simulink model "PFC_PID_Control_2_"  (R2025a)
settings: Solver=ode23tb  StartTime=0.0  StopTime=0.1  FixedStep=1e-06  MaxStep=1e-5  RelTol=1e-4  AbsTol=1e-6
undefined symbols (not defined in the file or in its folder): I_pk
libraries: slpidlib x2
settings Model: Creator=kesav  LastModifiedBy=kesav

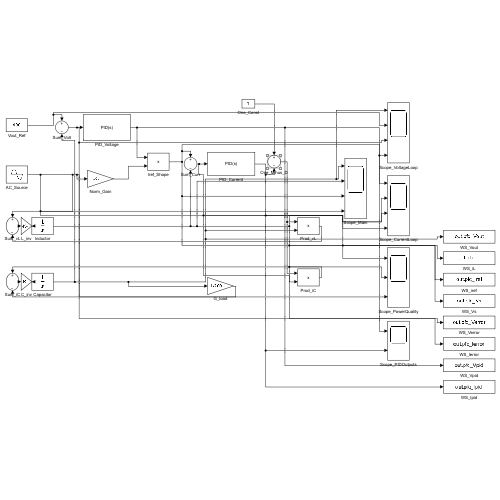
[thumbnail: Simulink's stored preview of the top-level diagram]
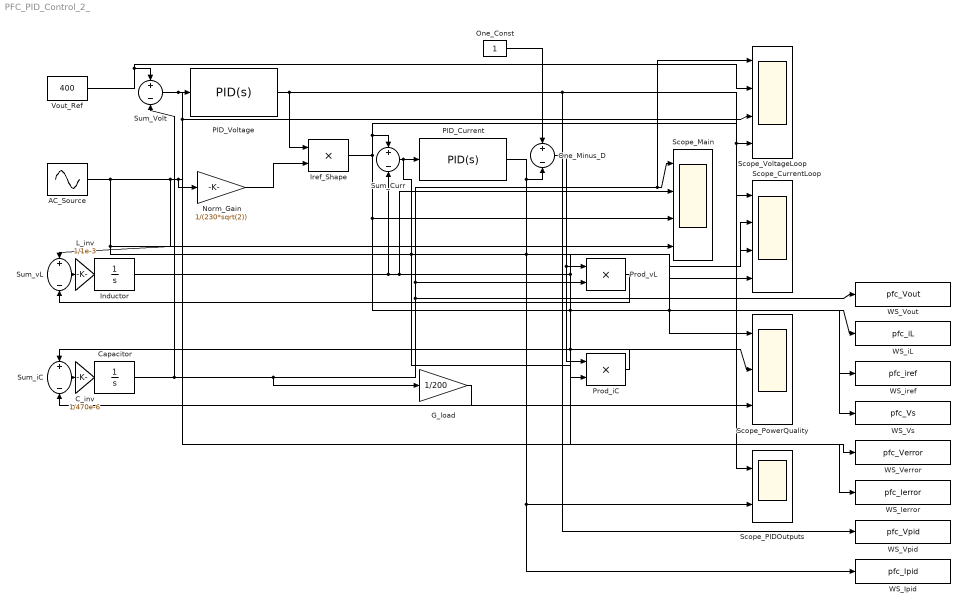
== system PFC_PID_Control_2_ ==
  AC_Source : Sin  Amplitude=325.27  Frequency=2*pi*50  SampleTime=0
  C_inv : Gain  Gain=1/470e-6
  Capacitor : Integrator
  G_load : Gain  Gain=1/200
  Inductor : Integrator
  Iref_Shape : Product
  L_inv : Gain  Gain=1/1e-3
  Norm_Gain : Gain  Gain=1/(230*sqrt(2))
  One_Const : Constant
  One_Minus_D : Sum  Inputs=+-
  PID_Current : slpidlib/PID Controller  Controller=PID  Form=Parallel  TimeDomain=Continuous-time  UseExternalTs=off  SampleTime=-1  IntegratorMethod=Forward Euler  FilterMethod=Forward Euler  ControllerParametersSource=internal  P=0.5  I=50  UseKiTs=off  D=0  UseExternalDerivativeSource=off  N=100  UseFilter=on  TunerSelectOption=Transfer Function Based (PID Tuner App)  InitialConditionSource=internal  InitialConditionForIntegrator=0  InitialConditionForFilter=0  DifferentiatorICPrevScaledInput=0  ExternalReset=none  TrackingMode=off  Kt=1  LimitOutput=off  SatLimitsSource=internal  UpperSaturationLimit=0.95  LowerSaturationLimit=-0.95  LinearizeAsGain=on  AntiWindupMode=clamping  Kb=1  LimitIntegrator=off  UpperIntegratorSaturationLimit=inf  LowerIntegratorSaturationLimit=-inf  POutMin=[]  POutMax=[]  IOutMin=[]  IOutMax=[]  DOutMin=[]  DOutMax=[]  NOutMin=[]  NOutMax=[]  SumOutMin=[]  SumOutMax=[]  SaturationOutMin=[]  SaturationOutMax=[]  PParamMin=[]  PParamMax=[]  IParamMin=[]  IParamMax=[]  DParamMin=[]  DParamMax=[]  NParamMin=[]  NParamMax=[]  KbParamMin=[]  KbParamMax=[]  KtParamMin=[]  KtParamMax=[]  KbOutMin=[]  KbOutMax=[]  KtOutMin=[]  KtOutMax=[]  IntegratorOutMin=[]  IntegratorOutMax=[]  FilterOutMin=[]  FilterOutMax=[]  SumI1OutMin=[]  SumI1OutMax=[]  SumI2OutMin=[]  SumI2OutMax=[]  SumI3OutMin=[]  SumI3OutMax=[]  SumI4OutMin=[]  SumI4OutMax=[]  SumDOutMin=[]  SumDOutMax=[]  DifferentiatorOutMin=[]  DifferentiatorOutMax=[]  FilterDiffOutCoefMin=[]  FilterDiffOutCoefMax=[]  ReciprocalOutMin=[]  ReciprocalOutMax=[]  SumDenOutMin=[]  SumDenOutMax=[]  SumNumOutMin=[]  SumNumOutMax=[]  DivideOutMin=[]  DivideOutMax=[]  UdiffTsProdOutMin=[]  UdiffTsProdOutMax=[]  NTsProdOutMin=[]  NTsProdOutMax=[]  UintegralTsProdOutMin=[]  UintegralTsProdOutMax=[]  UngainTsProdOutMin=[]  UngainTsProdOutMax=[]  ClampingZeroOutDataTypeStr=Inherit: Inherit via back propagation  ClampingZeroOutMin=[]  ClampingZeroOutMax=[]  FilterDenConstantOutDataTypeStr=Inherit: Inherit via back propagation  FilterDenConstantOutMin=[]  FilterDenConstantOutMax=[]  PCopyOutDataTypeStr=Inherit: Inherit via back propagation  PCopyOutMin=[]  PCopyOutMax=[]  NCopyOutDataTypeStr=Inherit: Inherit via back propagation  NCopyOutMin=[]  NCopyOutMax=[]  IntegratorContinuousStateAttributes=''  IntegratorStateMustResolveToSignalObject=off  IntegratorRTWStateStorageClass=Auto  FilterContinuousStateAttributes=''  FilterStateMustResolveToSignalObject=off  FilterRTWStateStorageClass=Auto  ParallelPVariant=InternalParameters  IdealPVariant=Disabled  IVariant=InternalParameters  DVariant=InternalParameters  IntegratorVariant=Continuous  SatVariant=Disabled  AWVariant=Passthrough  PCopyVariant=Disabled  TRVariant=Disabled  FdbkBlocksVariant=Forward  IdealPFdbkVariant=Disabled  SatFdbkVariant=Disabled  DerivativeFilterVariant=ContFilter  NVariant=InternalParameters  NCopyVariant=Disabled  FilterICVariant=InternalICsFilter  IntegratorICVariant=InternalICs  ExternalResetVariant=Disabled  TRSumVariant=Passthrough  SumFdbkVariant=Disabled  SumVariant=Sum_PID  TsampFilterVariant=InternalTs  TsampNgainVariant=Passthrough  TsampIntegralVariant=Disabled_SignalSpec  ExternalSaturationOutDataTypeStr=Inherit: Same as second input  DerivativeSourceVariant=ErrorSignal  PreIntVariant=InternalPreInt
  PID_Voltage : slpidlib/PID Controller  Controller=PID  Form=Parallel  TimeDomain=Continuous-time  UseExternalTs=off  SampleTime=-1  IntegratorMethod=Forward Euler  FilterMethod=Forward Euler  ControllerParametersSource=internal  P=0.3  I=20  UseKiTs=off  D=0  UseExternalDerivativeSource=off  N=10  UseFilter=on  TunerSelectOption=Transfer Function Based (PID Tuner App)  InitialConditionSource=internal  InitialConditionForIntegrator=0  InitialConditionForFilter=0  DifferentiatorICPrevScaledInput=0  ExternalReset=none  TrackingMode=off  Kt=1  LimitOutput=off  SatLimitsSource=internal  UpperSaturationLimit=I_pk  LowerSaturationLimit=0  LinearizeAsGain=on  AntiWindupMode=clamping  Kb=1  LimitIntegrator=off  UpperIntegratorSaturationLimit=inf  LowerIntegratorSaturationLimit=-inf  POutMin=[]  POutMax=[]  IOutMin=[]  IOutMax=[]  DOutMin=[]  DOutMax=[]  NOutMin=[]  NOutMax=[]  SumOutMin=[]  SumOutMax=[]  SaturationOutMin=[]  SaturationOutMax=[]  PParamMin=[]  PParamMax=[]  IParamMin=[]  IParamMax=[]  DParamMin=[]  DParamMax=[]  NParamMin=[]  NParamMax=[]  KbParamMin=[]  KbParamMax=[]  KtParamMin=[]  KtParamMax=[]  KbOutMin=[]  KbOutMax=[]  KtOutMin=[]  KtOutMax=[]  IntegratorOutMin=[]  IntegratorOutMax=[]  FilterOutMin=[]  FilterOutMax=[]  SumI1OutMin=[]  SumI1OutMax=[]  SumI2OutMin=[]  SumI2OutMax=[]  SumI3OutMin=[]  SumI3OutMax=[]  SumI4OutMin=[]  SumI4OutMax=[]  SumDOutMin=[]  SumDOutMax=[]  DifferentiatorOutMin=[]  DifferentiatorOutMax=[]  FilterDiffOutCoefMin=[]  FilterDiffOutCoefMax=[]  ReciprocalOutMin=[]  ReciprocalOutMax=[]  SumDenOutMin=[]  SumDenOutMax=[]  SumNumOutMin=[]  SumNumOutMax=[]  DivideOutMin=[]  DivideOutMax=[]  UdiffTsProdOutMin=[]  UdiffTsProdOutMax=[]  NTsProdOutMin=[]  NTsProdOutMax=[]  UintegralTsProdOutMin=[]  UintegralTsProdOutMax=[]  UngainTsProdOutMin=[]  UngainTsProdOutMax=[]  ClampingZeroOutDataTypeStr=Inherit: Inherit via back propagation  ClampingZeroOutMin=[]  ClampingZeroOutMax=[]  FilterDenConstantOutDataTypeStr=Inherit: Inherit via back propagation  FilterDenConstantOutMin=[]  FilterDenConstantOutMax=[]  PCopyOutDataTypeStr=Inherit: Inherit via back propagation  PCopyOutMin=[]  PCopyOutMax=[]  NCopyOutDataTypeStr=Inherit: Inherit via back propagation  NCopyOutMin=[]  NCopyOutMax=[]  IntegratorContinuousStateAttributes=''  IntegratorStateMustResolveToSignalObject=off  IntegratorRTWStateStorageClass=Auto  FilterContinuousStateAttributes=''  FilterStateMustResolveToSignalObject=off  FilterRTWStateStorageClass=Auto  ParallelPVariant=InternalParameters  IdealPVariant=Disabled  IVariant=InternalParameters  DVariant=InternalParameters  IntegratorVariant=Continuous  SatVariant=Disabled  AWVariant=Passthrough  PCopyVariant=Disabled  TRVariant=Disabled  FdbkBlocksVariant=Forward  IdealPFdbkVariant=Disabled  SatFdbkVariant=Disabled  DerivativeFilterVariant=ContFilter  NVariant=InternalParameters  NCopyVariant=Disabled  FilterICVariant=InternalICsFilter  IntegratorICVariant=InternalICs  ExternalResetVariant=Disabled  TRSumVariant=Passthrough  SumFdbkVariant=Disabled  SumVariant=Sum_PID  TsampFilterVariant=InternalTs  TsampNgainVariant=Passthrough  TsampIntegralVariant=Disabled_SignalSpec  ExternalSaturationOutDataTypeStr=Inherit: Same as second input  DerivativeSourceVariant=ErrorSignal  PreIntVariant=InternalPreInt
  Prod_iC : Product
  Prod_vL : Product
  Scope_CurrentLoop : Scope  NumInputPorts=4
      settings: ActiveDisplayYMinimum=-45.830688238369063  ActiveDisplayYMaximum=53.057681548956552
  Scope_Main : Scope  NumInputPorts=4
  Scope_PIDOutputs : Scope  NumInputPorts=2
      settings: ActiveDisplayYMinimum=-1  ActiveDisplayYMaximum=1
  Scope_PowerQuality : Scope  NumInputPorts=3
      settings: ActiveDisplayYMinimum=-1  ActiveDisplayYMaximum=1
  Scope_VoltageLoop : Scope  NumInputPorts=4
  Sum_Curr : Sum  Inputs=+-
  Sum_Volt : Sum  Inputs=+-
  Sum_iC : Sum  Inputs=+-
  Sum_vL : Sum  Inputs=+-
  Vout_Ref : Constant  Value=400
  WS_Ierror : ToWorkspace  VariableName=pfc_Ierror  SampleTime=-1
  WS_Ipid : ToWorkspace  VariableName=pfc_Ipid  SampleTime=-1
  WS_Verror : ToWorkspace  VariableName=pfc_Verror  SampleTime=-1
  WS_Vout : ToWorkspace  VariableName=pfc_Vout  SampleTime=-1
  WS_Vpid : ToWorkspace  VariableName=pfc_Vpid  SampleTime=-1
  WS_Vs : ToWorkspace  VariableName=pfc_Vs  SampleTime=-1
  WS_iL : ToWorkspace  VariableName=pfc_iL  SampleTime=-1
  WS_iref : ToWorkspace  VariableName=pfc_iref  SampleTime=-1
  wires:
  Vout_Ref/1 -> Sum_Volt/1, Scope_VoltageLoop/2
  AC_Source/1 -> Norm_Gain/1, Scope_PowerQuality/3, Sum_vL/1, Scope_PowerQuality/1, WS_Vs/1, Scope_Main/4
  PID_Voltage/1 -> Scope_VoltageLoop/4, Scope_PIDOutputs/1, WS_Vpid/1, Iref_Shape/1
  Norm_Gain/1 -> Iref_Shape/2
  Iref_Shape/1 -> Scope_Main/3, WS_iref/1, Sum_Curr/1, Scope_CurrentLoop/1
  Prod_vL/1 -> Sum_vL/2
  Sum_vL/1 -> L_inv/1
  L_inv/1 -> Inductor/1
  Prod_iC/1 -> Sum_iC/1
  G_load/1 -> Sum_iC/2
  Sum_iC/1 -> C_inv/1
  C_inv/1 -> Capacitor/1
  One_Const/1 -> One_Minus_D/1
  PID_Current/1 -> Scope_PIDOutputs/2, WS_Ipid/1, Scope_CurrentLoop/4, One_Minus_D/2
  Inductor/1 -> Sum_Curr/2, Prod_iC/2, Scope_PowerQuality/2, WS_iL/1, Scope_CurrentLoop/2, Scope_Main/2
  One_Minus_D/1 -> Prod_vL/1, Prod_iC/1
  Capacitor/1 -> Scope_Main/1, Scope_VoltageLoop/1, Prod_vL/2, WS_Vout/1, G_load/1, Sum_Volt/2
  Sum_Volt/1 -> Scope_VoltageLoop/3, WS_Verror/1, PID_Voltage/1
  Sum_Curr/1 -> PID_Current/1, Scope_CurrentLoop/3, WS_Ierror/1
